simulink model "inverter_power_model"  (R2026a)
settings: Solver=VariableStepAuto
PreLoadFcn:
  | run(fullfile(pwd,'data','inverter_efficiency_map.m'))
undefined symbols (not defined in the file): I_ac_bp, P_loss_table, V_dc_bp
settings Model: Creator=golov  LastModifiedBy=renil

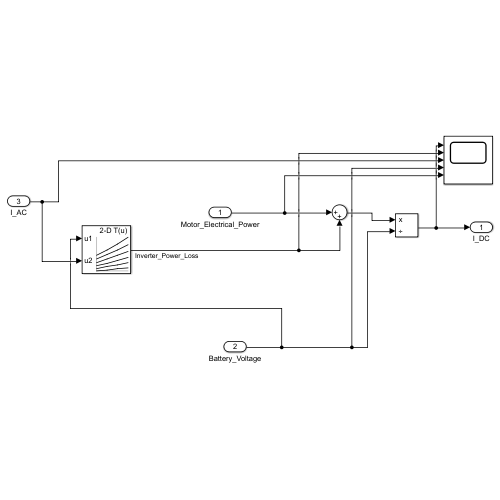
[thumbnail: Simulink's stored preview of the top-level diagram]
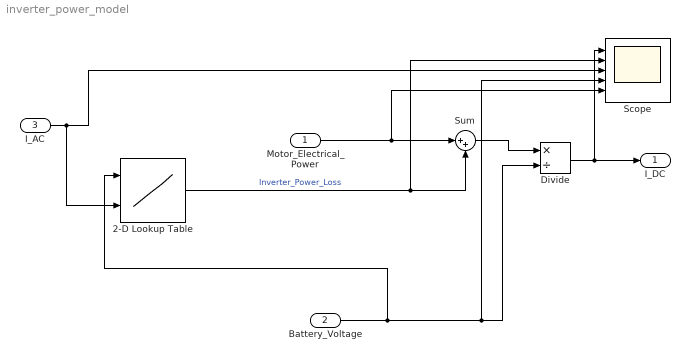
== system inverter_power_model ==
  Motor_Electrical_Power : Inport
  Battery_Voltage : Inport  Port=2
  I_AC : Inport  Port=3
  2-D Lookup Table : Lookup_n-D  BreakpointsForDimension1=V_dc_bp  BreakpointsForDimension2=I_ac_bp  Table=P_loss_table  InternalRulePriority=Speed  RndMeth=Simplest
      settings: InputPortMap=u0,u1
  Divide : Product  Inputs=*/
  Scope : Scope  NumInputPorts=5
      settings: ActiveDisplayYMinimum=-141.8246963681587  ActiveDisplayYMaximum=256.19846303454642
  Sum : Sum  Inputs=|++
  I_DC : Outport
  wires:
  Battery_Voltage/1 -> 2-D Lookup Table/1, Scope/4, Divide/2
  Divide/1 -> Scope/1, I_DC/1
  Sum/1 -> Divide/1
  Motor_Electrical_Power/1 -> Scope/5, Sum/1
  2-D Lookup Table/1 -> Scope/2, Sum/2  "Inverter_Power_Loss"
  I_AC/1 -> 2-D Lookup Table/2, Scope/3
